simulink model "TV_Thermal_4WD"  (R2024b)
settings: Solver=VariableStepAuto  StartTime=0.0  StopTime=10.0  RelTol=1e-3
settings Model: Creator=nikil  LastModifiedBy=nikil

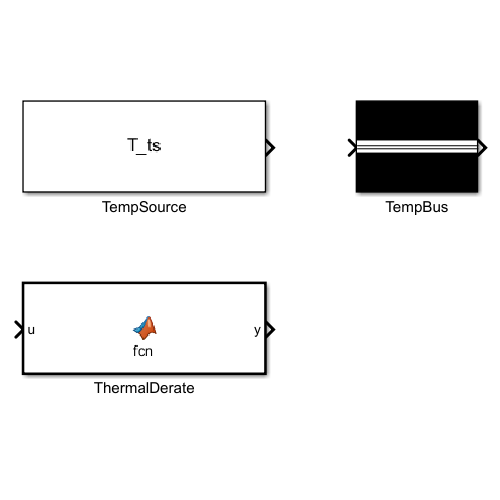
[thumbnail: Simulink's stored preview of the top-level diagram]
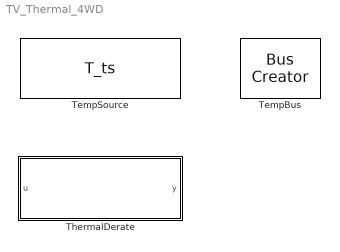
== system TV_Thermal_4WD ==
  TempBus : BusCreator  Inputs=1
  TempSource : FromWorkspace  VariableName=T_ts  SampleTime=-1
  ThermalDerate : MATLAB Function  TreatAsAtomicUnit=on

== matlab function TV_Thermal_4WD/ThermalDerate ==
  data: u input; y output
function y = fcn(u)

y = u;
